simulink model "Control1DOF"  (R2024b)
settings: Solver=VariableStepAuto  StartTime=0.0  StopTime=10.0  RelTol=1e-3
undefined symbols (not defined in the file or in its folder): a
settings Model: Creator=crazy  LastModifiedBy=crazy

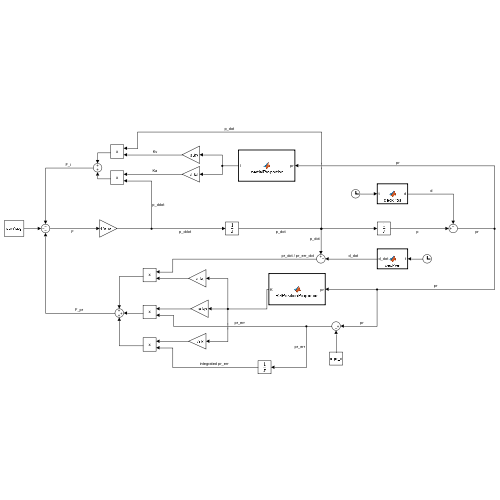
[thumbnail: Simulink's stored preview of the top-level diagram]
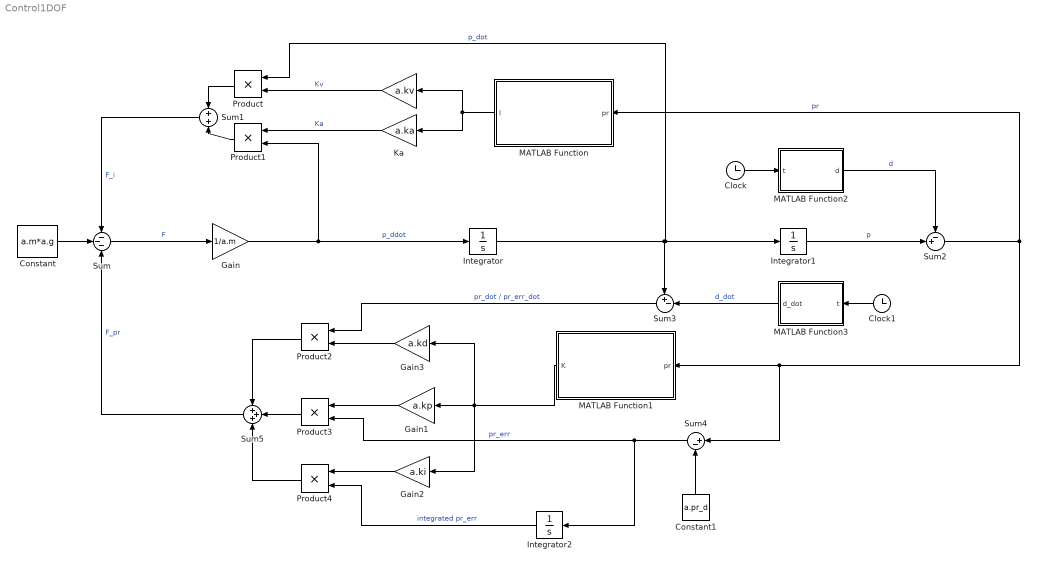
== system Control1DOF ==
  " " : Gain  Gain=a.kv
  Clock : Clock
  Clock1 : Clock
  Constant : Constant  Value=a.m*a.g
  Constant1 : Constant  Value=a.pr_d
  Gain : Gain  Gain=1/a.m
  Gain1 : Gain  Gain=a.kp
  Gain2 : Gain  Gain=a.ki
  Gain3 : Gain  Gain=a.kd
  Integrator : Integrator  InitialCondition=a.d_dot(0)
  Integrator1 : Integrator  InitialCondition=a.d(0)+a.pr_d
  Integrator2 : Integrator
  Ka : Gain  Gain=a.ka
  MATLAB Function : MATLAB Function  TreatAsAtomicUnit=on
  MATLAB Function1 : MATLAB Function  TreatAsAtomicUnit=on
  MATLAB Function2 : MATLAB Function  TreatAsAtomicUnit=on
  MATLAB Function3 : MATLAB Function  TreatAsAtomicUnit=on
  Product{,1..4} (5 alike) : Product
  Sum : Sum  Inputs=---
  Sum1 : Sum  Inputs=+|+
  Sum2 : Sum  Inputs=-+|
  Sum3 : Sum  Inputs=+-|
  Sum4 : Sum  Inputs=|+-
  Sum5 : Sum  Inputs=+++
  wires:
  Gain/1 -> Product1/2, Integrator/1  "p_ddot"
  Integrator/1 -> Integrator1/1, Product/1, Sum3/1  "p_dot"
  Sum/1 -> Gain/1  "F"
  Integrator1/1 -> Sum2/2  "p"
  MATLAB Function/1(I) -> " "/1, Ka/1
  Ka/1 -> Product1/1  "Ka"
  " "/1 -> Product/2  "Kv"
  Product/1 -> Sum1/1
  Product1/1 -> Sum1/2
  Sum1/1 -> Sum/1  "F_i"
  Constant/1 -> Sum/2
  MATLAB Function2/1(d) -> Sum2/1  "d"
  Sum2/1 -> Sum4/1, MATLAB Function1/1(pr), MATLAB Function/1(pr)  "pr"
  Clock/1 -> MATLAB Function2/1(t)
  Clock1/1 -> MATLAB Function3/1(t)
  MATLAB Function3/1(d_dot) -> Sum3/2  "d_dot"
  MATLAB Function1/1(K) -> Gain3/1, Gain1/1, Gain2/1
  Gain1/1 -> Product3/1
  Gain3/1 -> Product2/2
  Gain2/1 -> Product4/1
  Integrator2/1 -> Product4/2  "integrated pr_err"
  Constant1/1 -> Sum4/2
  Sum4/1 -> Integrator2/1, Product3/2  "pr_err"
  Sum3/1 -> Product2/1  "pr_dot / pr_err_dot"
  Product3/1 -> Sum5/2
  Product2/1 -> Sum5/1
  Product4/1 -> Sum5/3
  Sum5/1 -> Sum/3  "F_pr"

== matlab function Control1DOF/MATLAB Function ==
  data: pr input; I output
function I = InertialProportion(pr)

I = a.I(pr);

== matlab function Control1DOF/MATLAB Function2 ==
  data: t input; d output
function d = deckPos(t)

d = a.d(t);

== matlab function Control1DOF/MATLAB Function3 ==
  data: t input; d_dot output
function d_dot = deckVel(t)

d_dot = a.d_dot(t);

== matlab function Control1DOF/MATLAB Function1 ==
  data: pr input; K output
function K = RelPositionProportion(pr)

K = a.K(pr);
